simulink model "ACCAEB4_1"  (R2015a)
settings: Solver=ode3  StartTime=0.0  StopTime=10  FixedStep=0.1  RelTol=1e-3
undefined symbols (not defined in the file): aAEB, AbsAccMax, AEBTTCInput, g, HeadwayTime_desire, Kpid, rAEB, RLIni, RMin, RoadFrictionCoeff, StopWhenAEBOn, Ts, vIni
libraries: simulink x2
settings Model: CovSFcnEnable=off  Creator=Ding Zhao  LastModifiedBy=zhaoding
settings DataIOCC: LimitDataPoints=off  SaveOutput=off
settings OptimizationCC: ExpressionDepthLimit=2147483647
settings DebuggingCC: UnderspecifiedInitializationDetection=Classic  MergeDetectMultiDrivingBlocksExec=none  SolverPrmCheckMsg=warning  FcnCallInpInsideContextMsg=UseLocalSettings  StateNameClashWarn=warning
settings GRTTargetCC: CombineOutputUpdateFcns=off  GRTInterface=on

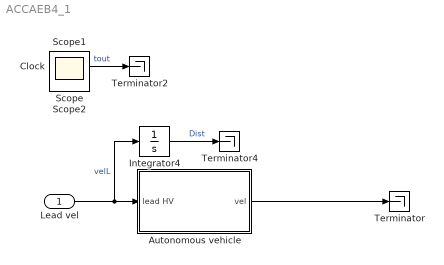
== system ACCAEB4_1 ==
  Lead vel : Inport
  Autonomous vehicle : Subsystem
  Clock : Clock
  Integrator4 : Integrator
  Terminator : Terminator
  Terminator2 : Terminator
  Terminator4 : Terminator
  Scope : Scope  NumInputPorts=4
      settings: ShowLegends=on  TimeRange=9  YMin=-5~-10~10~-5  YMax=40~4~35~3  MaxDataPoints=7500
  Scope1 : Scope  NumInputPorts=2
      settings: YMin=-5~-5  YMax=5~5  MaxDataPoints=7500
  Scope2 : Scope  NumInputPorts=4
      settings: ShowLegends=on  YMin=-5~-5~-5~-5  YMax=5~5~5~5  SaveName=ScopeData2  MaxDataPoints=7500
  wires:
  Autonomous vehicle/1(vel) -> Terminator/1
  Clock/1 -> Terminator2/1  "tout"
  Lead vel/1 -> Integrator4/1, Autonomous vehicle/1(lead HV)  "velL"
  Integrator4/1 -> Terminator4/1  "Dist"

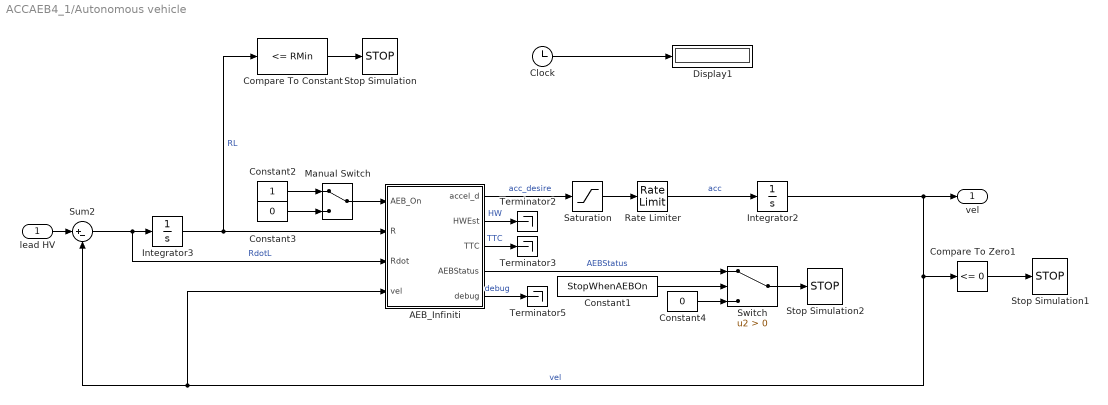
== system ACCAEB4_1/Autonomous vehicle ==
  lead HV : Inport
  AEB_Infiniti : MATLAB Function  TreatAsAtomicUnit=on  SystemSampleTime=Ts
  Clock : Clock
  Compare To Constant : simulink/Logic and Bit Operations/Compare To Constant  relop=<=  const=RMin  OutDataTypeStr=boolean
  Compare To Zero1 : simulink/Logic and Bit Operations/Compare To Zero  relop=<=  OutDataTypeStr=boolean
  Constant1 : Constant  Value=StopWhenAEBOn  SampleTime=Ts
  Constant2 : Constant  SampleTime=Ts
  Constant3 : Constant  Value=0  SampleTime=Ts
  Constant4 : Constant  Value=0  SampleTime=Ts
  Display1 : Display
  Integrator2 : Integrator  InitialCondition=vIni  LowerSaturationLimit=0
  Integrator3 : Integrator  InitialCondition=RLIni
  Manual Switch : ManualSwitch
  Rate Limiter : RateLimiter  RisingSlewLimit=20  FallingSlewLimit=-20  SampleTimeMode=inherited
  Saturation : Saturate  UpperLimit=RoadFrictionCoeff*g  LowerLimit=-RoadFrictionCoeff*g
  Stop Simulation : Stop
  Stop Simulation1 : Stop
  Stop Simulation2 : Stop
  Sum2 : Sum  Inputs=|+-
  Switch : Switch  Criteria=u2 > Threshold
  Terminator2 : Terminator
  Terminator3 : Terminator
  Terminator5 : Terminator
  vel : Outport
  wires:
  AEB_Infiniti/1(accel_d) -> Saturation/1  "acc_desire"
  Sum2/1 -> AEB_Infiniti/3(Rdot), Integrator3/1  "RdotL"
  Integrator3/1 -> Compare To Constant/1, AEB_Infiniti/2(R)  "RL"
  Saturation/1 -> Rate Limiter/1
  Compare To Constant/1 -> Stop Simulation/1
  lead HV/1 -> Sum2/1
  AEB_Infiniti/2(HWEst) -> Terminator2/1  "HW"
  AEB_Infiniti/3(TTC) -> Terminator3/1  "TTC"
  Manual Switch/1 -> AEB_Infiniti/1(AEB_On)
  Constant2/1 -> Manual Switch/1
  Constant3/1 -> Manual Switch/2
  AEB_Infiniti/4(AEBStatus) -> Switch/1  "AEBStatus"
  AEB_Infiniti/5(debug) -> Terminator5/1  "debug"
  Clock/1 -> Display1/1
  Integrator2/1 -> AEB_Infiniti/4(vel), Sum2/2, Compare To Zero1/1, vel/1  "vel"
  Compare To Zero1/1 -> Stop Simulation1/1
  Rate Limiter/1 -> Integrator2/1  "acc"
  Switch/1 -> Stop Simulation2/1
  Constant1/1 -> Switch/2
  Constant4/1 -> Switch/3

== matlab function ACCAEB4_1/Autonomous vehicle/AEB_Infiniti ==
  data: AEB_On input; HeadwayTime_desire parameter; R input; Rdot input; accel_d output; vel input; Kpid parameter; HWEst output; TTC output; AEBStatus output; debug output; rAEB parameter; aAEB parameter; AEBTTCInput parameter; AbsAccMax parameter
function [accel_d,HWEst,TTC,AEBStatus,debug] = fcn(AEB_On, HeadwayTime_desire,R,Rdot,vel,Kpid,rAEB,aAEB,AEBTTCInput,AbsAccMax)
%#codegen
persistent HWErr AEBFlag accLog AEBTimer AEBIniAcc
if isempty(HWErr), HWErr = 0;end;
if isempty(AEBFlag), AEBFlag = 0;end;
if isempty(accLog), accLog = 0;end;
if isempty(AEBTimer), AEBTimer = 0;end;
if isempty(AEBIniAcc), AEBIniAcc = 0;end;
HWErrLast = HWErr;
AEBFlagLast = AEBFlag;
Ts = 0.1; % sampling time
HW_d = HeadwayTime_desire;
%% ACC setting
HWEst = R/vel;
HWErr = HW_d - HWEst;
Kp = Kpid(1);
Ki = Kpid(2);
% Kd = Kpid(3);
accMax = AbsAccMax;
accMin = -AbsAccMax;

%% AEB setting
% VelLead = Rdot-vel; Rdot-vel
TTC = -R/Rdot;
TTC_AEBRelease = 1;


%% AEB trigger
% AEBTTCInput = [    4.1667   11.1111;
%                    0.8579    0.9100;
%                    0.0075         0];

if isempty(find(AEBTTCInput(1,:)<=vel,1,'last'))
    fprintf('PieceInd is empty');
    PieceInd= 1;
else
    PieceInd = min(find(AEBTTCInput(1,:)<=vel,1,'last'));
end
    
TTC_AEB = AEBTTCInput(2,PieceInd)+AEBTTCInput(3,PieceInd)*(vel-AEBTTCInput(1,PieceInd));
% if isempty(PieceInd)
%     fprintf('PieceInd is empty');
%     PieceInd= 1;
% end
if TTC > 0 && TTC <= TTC_AEB && AEB_On == 1
    AEBFlag = 1;
elseif TTC > TTC_AEBRelease || TTC < 0
    AEBFlag = 0;
end
debug = [AEBFlagLast;AEBFlag;HWErrLast];
AEBStatus = AEBFlag;
%% control
if AEBFlag == 0
    if AEBFlagLast == 1
        HWErrLast = 0;
        AEBTimer = 0;
    end
    accel_d = accLog+Kp*(HWErr-HWErrLast)+Ki*Ts/2*(HWErr+HWErrLast); % pi controller
    if vel >= 90/2.236 && accel_d > 0 % 70 mph speed limit
        accel_d = 0;
    else
        accel_d = max(min(accel_d,accMax),accMin);
    end
else
    if AEBFlagLast == 0
        AEBIniAcc = accLog;
    end
    AEBTimer = AEBTimer + 0.1;
    accel_d = AEBIniAcc + AEBTimer*rAEB;
    accel_d = max(aAEB,accel_d);
%     debug = [0,0,0];
end
accLog = accel_d;
